simulink model "week3problem3"  (R2020b)
settings: Solver=VariableStepAuto  StartTime=0.0  StopTime=10.0  RelTol=1e-3
settings Model: Creator=HP  LastModifiedBy=HP

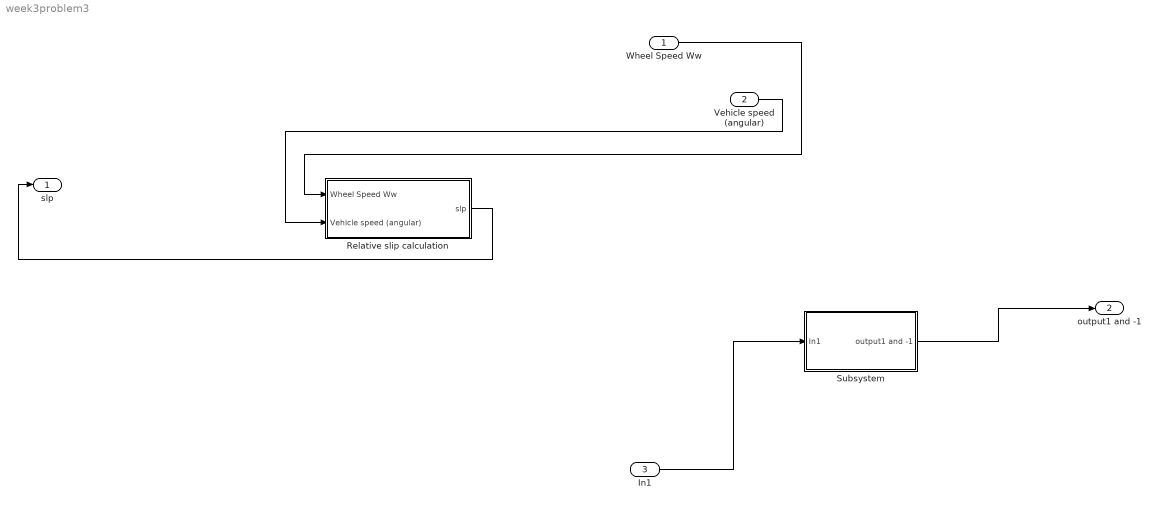
== system week3problem3 ==
  Wheel Speed Ww : Inport
  Vehicle speed (angular) : Inport  Port=2
  In1 : Inport  Port=3
  Relative slip calculation : Subsystem
  Subsystem : Subsystem
  slp : Outport
  output1 and -1 : Outport  Port=2
  wires:
  Wheel Speed Ww/1 -> Relative slip calculation/1(Wheel Speed Ww)
  Vehicle speed (angular)/1 -> Relative slip calculation/2(Vehicle speed (angular))
  Relative slip calculation/1(slp) -> slp/1
  In1/1 -> Subsystem/1(In1)
  Subsystem/1(output1 and -1) -> output1 and -1/1

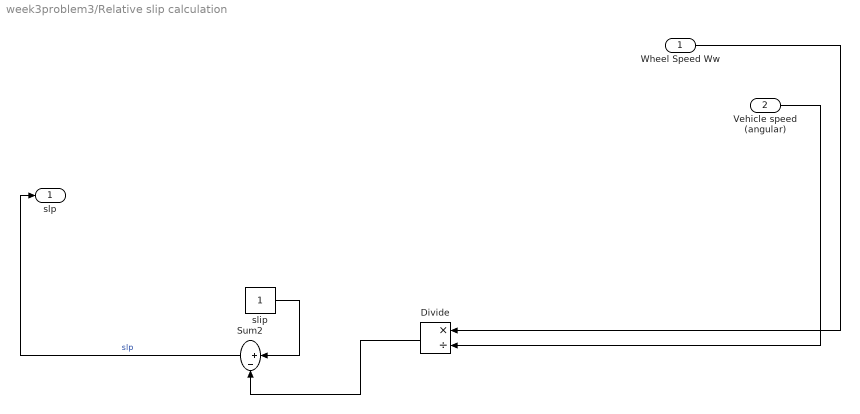
== system week3problem3/Relative slip calculation ==
  Wheel Speed Ww : Inport
  Vehicle speed (angular) : Inport  Port=2
  Divide : Product  Inputs=*/
  Sum2 : Sum  Inputs=|+-  InputSameDT=on  SaturateOnIntegerOverflow=on  OutDataTypeStr=Inherit: Same as first input
  slip : Constant
  slp : Outport
  wires:
  slip/1 -> Sum2/1
  Sum2/1 -> slp/1  "slp"
  Wheel Speed Ww/1 -> Divide/1
  Vehicle speed (angular)/1 -> Divide/2
  Divide/1 -> Sum2/2

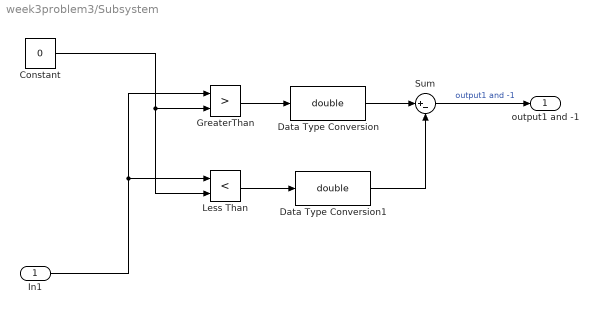
== system week3problem3/Subsystem ==
  In1 : Inport
  Constant : Constant  Value=0
  Data Type Conversion : DataTypeConversion  OutDataTypeStr=double  RndMeth=Zero
  Data Type Conversion1 : DataTypeConversion  OutDataTypeStr=double  RndMeth=Zero
  GreaterThan : RelationalOperator  Operator=>  OutDataTypeStr=boolean  RndMeth=Simplest
  Less Than : RelationalOperator  Operator=<  OutDataTypeStr=boolean  RndMeth=Simplest
  Sum : Sum  Inputs=|+-
  output1 and -1 : Outport
  wires:
  GreaterThan/1 -> Data Type Conversion/1
  Less Than/1 -> Data Type Conversion1/1
  Constant/1 -> Less Than/2, GreaterThan/2
  Sum/1 -> output1 and -1/1  "output1 and -1"
  In1/1 -> Less Than/1, GreaterThan/1
  Data Type Conversion/1 -> Sum/1
  Data Type Conversion1/1 -> Sum/2
